simulink model "test_kalman_pitch"  (R2023b)
settings: Solver=VariableStepAuto  StartTime=0.0  StopTime=15  RelTol=1e-3
values from neighbouring files (symbols this model uses):
  A = [0.0, -1.0; 0.0, 0.0]    [calcKalmanGain_pitch_bias.m]    (also in calcKalmanGain_pitch_only.m = 0; compFilter.m = [0 -1; 0  0])
  B = [1.0 ... (first row only)    [calcKalmanGain_pitch_bias.m]    (also in calcKalmanGain_pitch_only.m = 1; compFilter.m = [1; 0])
  C = [1.0, 0.0]    [calcKalmanGain_pitch_bias.m]    (also in calcKalmanGain_pitch_only.m = 1; compFilter.m = [1 0])
  D = [0]    [calcKalmanGain_pitch_bias.m]    (also in calcKalmanGain_pitch_only.m = 0; compFilter.m = 0)
  Lk = 0.316    [compFilter.m]
libraries: simulink x2
settings Model: Creator=joaolehodey  LastModifiedBy=joaolehodey

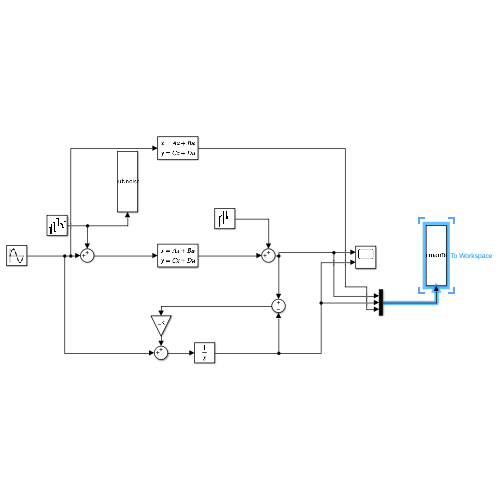
[thumbnail: Simulink's stored preview of the top-level diagram]
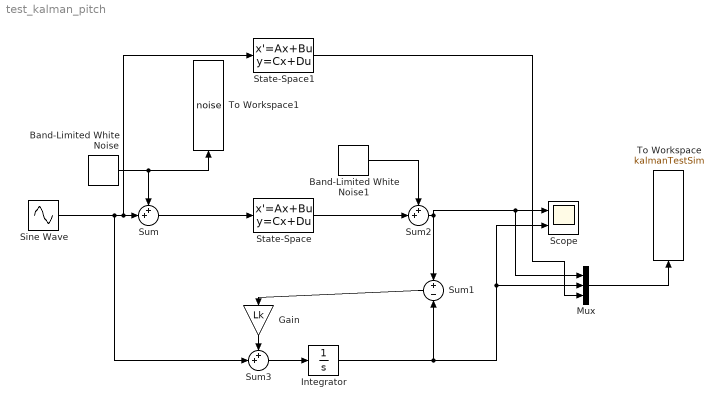
== system test_kalman_pitch ==
  Band-Limited White Noise : simulink/Sources/Band-Limited White Noise  Cov=[0.001]  Ts=0.005  seed=[241]
  Band-Limited White Noise1 : simulink/Sources/Band-Limited White Noise  Cov=[0.001]  Ts=0.005  seed=[245]
  Gain : Gain  Gain=Lk
  Integrator : Integrator  InitialCondition=-3
  Mux : Mux  Inputs=3
  Scope : Scope  NumInputPorts=2
  Sine Wave : Sin  SampleTime=0
  State-Space : StateSpace  A=A  B=B  C=C  D=D  InitialCondition=0
  State-Space1 : StateSpace  A=A  B=B  C=C  D=D  InitialCondition=0
  Sum : Sum  Inputs=++|
  Sum1 : Sum  Inputs=+|-
  Sum2 : Sum  Inputs=++|
  Sum3 : Sum  Inputs=++|
  To Workspace : ToWorkspace  VariableName=kalmanTestSim  SaveFormat=Timeseries  SampleTime=-1
  To Workspace1 : ToWorkspace  VariableName=noise  SaveFormat=Structure With Time  SampleTime=-1
  wires:
  Sine Wave/1 -> Sum3/2, State-Space1/1, Sum/2
  Band-Limited White Noise/1 -> To Workspace1/1, Sum/1
  Sum/1 -> State-Space/1
  Sum3/1 -> Integrator/1
  Sum1/1 -> Gain/1
  Band-Limited White Noise1/1 -> Sum2/1
  Sum2/1 -> Sum1/1, Mux/1, Scope/1
  Gain/1 -> Sum3/1
  Integrator/1 -> Mux/2, Scope/2, Sum1/2
  Mux/1 -> To Workspace/1
  State-Space/1 -> Sum2/2
  State-Space1/1 -> Mux/3
